simulink model "fcsystem"  (Simulink 5.0)
settings: Solver=ode23s  StartTime=0.0  StopTime=30.0  MaxStep=0.01  RelTol=1e-5
undefined symbols (not defined in the file or in its folder): alliedsignaleff, beta0, beta1, beta2, cm_kt, cm_kv, cm_maxtorque, cm_R, Cp, cp_inertia, dc, faradays, fc_activearea, fc_anode_volume, fc_cathode_volume, fc_inlet_flow_constant, fc_numberofcells, fc_outlet_flow_constant, fcx0, gamma, hydrogengasconstant, hydrogenmolarmass, im_volume, membranedrydensity, membranedryeqvweight, membranethickness, nitrogengasconstant, nitrogenmolarmass, om_At, om_Cd, om_outlet_choke_pr, om_volume, oxygengasconstant, oxygenmolarmass, phimax0, phimax1, phimax2, phimax3, phimax4, psimax0, psimax1, psimax2, psimax3, psimax4, psimax5, R, rho, Ta, universalgasconstant, vaporgasconstant, vapormolarmass
libraries: simulink x5
(part 2 of 3)

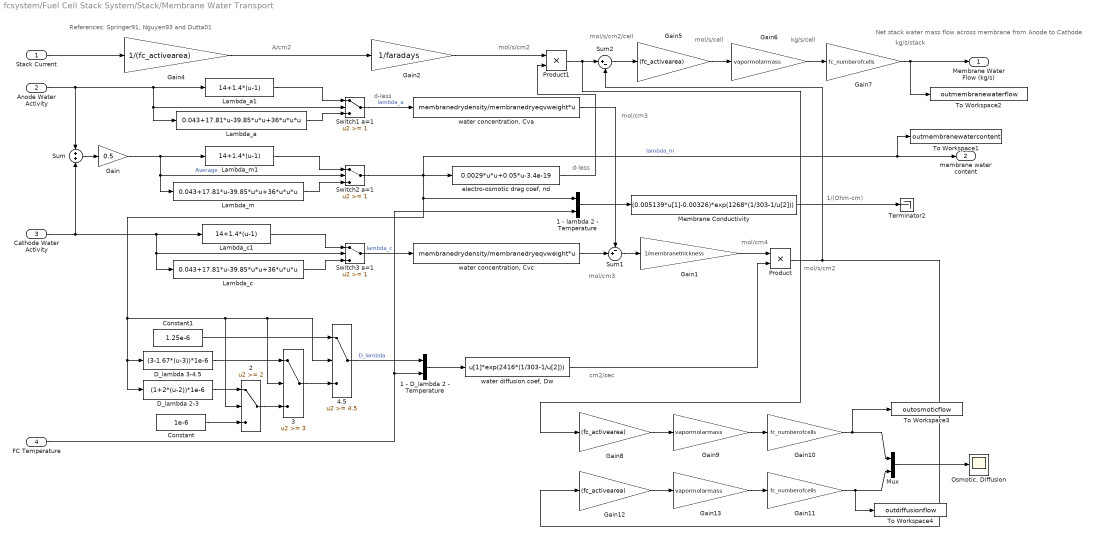
== system fcsystem/Fuel Cell Stack System/Stack/Membrane Water Transport ==
  note: kg/s/stack
  note: kg/s/cell
  note: mol/s/cell
  note: 1/(Ohm-cm)
  note: A/cm2
  note: mol/s/cm2/cell
  note: mol/s/cm2
  note: d-less
  note: mol/cm4
  note: cm2/sec
  note: mol/s/cm2
  note: mol/cm3
  note: mol/cm3
  note: d-less
  note: References: Springer91, Nguyen93 and Dutta01
  note: Net stack water mass flow
      | across membrane
      | from Anode to Cathode
  Stack Current : Inport
  Anode Water Activity : Inport  Port=2
  Cathode Water Activity : Inport  Port=3
  FC Temperature : Inport  Port=4
  1 - D_lambda 2 - Temperature : Mux  Inputs=2
  1 - lambda 2 - Temperature : Mux  Inputs=2
  2 : Switch  Threshold=2  SaturateOnIntegerOverflow=on  InputSameDT=on
  3 : Switch  Threshold=3  SaturateOnIntegerOverflow=on  InputSameDT=on
  4.5 : Switch  Threshold=4.5  SaturateOnIntegerOverflow=on  InputSameDT=on
  Constant : Constant  Value=1e-6
  Constant1 : Constant  Value=1.25e-6
  D_lambda 2-3 : Fcn  Expr=(1+2*(u-2))*1e-6
  D_lambda 3-4.5 : Fcn  Expr=(3-1.67*(u-3))*1e-6
  Gain : Gain  Gain=0.5  SaturateOnIntegerOverflow=on
  Gain1 : Gain  Gain=1/membranethickness  SaturateOnIntegerOverflow=on
  Gain10 : Gain  Gain=fc_numberofcells  SaturateOnIntegerOverflow=on
  Gain11 : Gain  Gain=fc_numberofcells  SaturateOnIntegerOverflow=on
  Gain12 : Gain  Gain=(fc_activearea)  SaturateOnIntegerOverflow=on
  Gain13 : Gain  Gain=vapormolarmass  SaturateOnIntegerOverflow=on
  Gain2 : Gain  Gain=1/faradays  SaturateOnIntegerOverflow=on
  Gain4 : Gain  Gain=1/(fc_activearea)  SaturateOnIntegerOverflow=on
  Gain5 : Gain  Gain=(fc_activearea)  SaturateOnIntegerOverflow=on
  Gain6 : Gain  Gain=vapormolarmass  SaturateOnIntegerOverflow=on
  Gain7 : Gain  Gain=fc_numberofcells  SaturateOnIntegerOverflow=on
  Gain8 : Gain  Gain=(fc_activearea)  SaturateOnIntegerOverflow=on
  Gain9 : Gain  Gain=vapormolarmass  SaturateOnIntegerOverflow=on
  Lambda_a : Fcn  Expr=0.043+17.81*u-39.85*u*u+36*u*u*u
  Lambda_a1 : Fcn  Expr=14+1.4*(u-1)
  Lambda_c : Fcn  Expr=0.043+17.81*u-39.85*u*u+36*u*u*u
  Lambda_c1 : Fcn  Expr=14+1.4*(u-1)
  Lambda_m : Fcn  Expr=0.043+17.81*u-39.85*u*u+36*u*u*u
  Lambda_m1 : Fcn  Expr=14+1.4*(u-1)
  Membrane Conductivity : Fcn  Expr=(0.005139*u[1]-0.00326)*exp(1268*(1/303-1/u[2]))
  Mux : Mux  Inputs=2
  "Osmotic, Diffusion" : Scope
      settings: TimeRange=15  YMin=0  YMax=0.02
  Product : Product  SaturateOnIntegerOverflow=on  InputSameDT=on
  Product1 : Product  SaturateOnIntegerOverflow=on  InputSameDT=on
  Sum : Sum  Inputs=+|+  SaturateOnIntegerOverflow=on  InputSameDT=on
  Sum1 : Sum  Inputs=-+|  SaturateOnIntegerOverflow=on  InputSameDT=on
  Sum2 : Sum  Inputs=|+-  SaturateOnIntegerOverflow=on  InputSameDT=on
  Switch1 a=1 : Switch  Threshold=1  SaturateOnIntegerOverflow=on  InputSameDT=on
  Switch2 a=1 : Switch  Threshold=1  SaturateOnIntegerOverflow=on  InputSameDT=on
  Switch3 a=1 : Switch  Threshold=1  SaturateOnIntegerOverflow=on  InputSameDT=on
  Terminator2 : Terminator
  To Workspace1 : ToWorkspace  VariableName=outmembranewatercontent  SampleTime=-1  SaveFormat=Array
  To Workspace2 : ToWorkspace  VariableName=outmembranewaterflow  SampleTime=-1  SaveFormat=Array
  To Workspace3 : ToWorkspace  VariableName=outosmoticflow  SampleTime=-1  SaveFormat=Array
  To Workspace4 : ToWorkspace  VariableName=outdiffusionflow  SampleTime=-1  SaveFormat=Array
  "electro-osmotic drag coef, nd" : Fcn  Expr=0.0029*u*u+0.05*u-3.4e-19
  "water concentration, Cva" : Fcn  Expr=membranedrydensity/membranedryeqvweight*u
  "water concentration, Cvc" : Fcn  Expr=membranedrydensity/membranedryeqvweight*u
  "water diffusion coef, Dw" : Fcn  Expr=u[1]*exp(2416*(1/303-1/u[2]))
  Membrane Water Flow (kg/s) : Outport
  membrane water content : Outport  Port=2
  wires:
  Gain11/1 -> To Workspace4/1, Mux/2
  Gain10/1 -> To Workspace3/1, Mux/1
  Gain7/1 -> To Workspace2/1, Membrane Water Flow (kg/s)/1
  Mux/1 -> "Osmotic, Diffusion"/1
  Product/1 -> Gain12/1, Sum2/2
  Gain13/1 -> Gain11/1
  Gain12/1 -> Gain13/1
  Gain9/1 -> Gain10/1
  Gain8/1 -> Gain9/1
  Product1/1 -> Gain8/1, Sum2/1
  Gain6/1 -> Gain7/1
  Gain5/1 -> Gain6/1
  Sum2/1 -> Gain5/1
  "electro-osmotic drag coef, nd"/1 -> Product1/2
  Gain2/1 -> Product1/1
  Gain4/1 -> Gain2/1
  Stack Current/1 -> Gain4/1
  1 - lambda 2 - Temperature/1 -> Membrane Conductivity/1
  FC Temperature/1 -> 1 - lambda 2 - Temperature/2, 1 - D_lambda 2 - Temperature/2
  Membrane Conductivity/1 -> Terminator2/1
  1 - D_lambda 2 - Temperature/1 -> "water diffusion coef, Dw"/1
  Gain1/1 -> Product/1
  "water diffusion coef, Dw"/1 -> Product/2
  Sum1/1 -> Gain1/1
  "water concentration, Cva"/1 -> Sum1/1
  "water concentration, Cvc"/1 -> Sum1/2
  Switch3 a=1/1 -> "water concentration, Cvc"/1  "lambda_c"
  Switch1 a=1/1 -> "water concentration, Cva"/1  "lambda_a"
  4.5/1 -> 1 - D_lambda 2 - Temperature/1  "D_lambda"
  Constant1/1 -> 4.5/1
  3/1 -> 4.5/3
  D_lambda 3-4.5/1 -> 3/1
  2/1 -> 3/3
  D_lambda 2-3/1 -> 2/1
  Lambda_c1/1 -> Switch3 a=1/1
  Lambda_c/1 -> Switch3 a=1/3
  Cathode Water Activity/1 -> Lambda_c/1, Switch3 a=1/2, Lambda_c1/1, Sum/2
  Constant/1 -> 2/3
  Switch2 a=1/1 -> To Workspace1/1, membrane water content/1, 1 - lambda 2 - Temperature/1, D_lambda 3-4.5/1, D_lambda 2-3/1, 2/2, 3/2, 4.5/2, "electro-osmotic drag coef, nd"/1  "lambda_m"
  Lambda_m/1 -> Switch2 a=1/3
  Lambda_m1/1 -> Switch2 a=1/1
  Gain/1 -> Lambda_m/1, Switch2 a=1/2, Lambda_m1/1  "Average"
  Sum/1 -> Gain/1
  Lambda_a/1 -> Switch1 a=1/3
  Lambda_a1/1 -> Switch1 a=1/1
  Anode Water Activity/1 -> Switch1 a=1/2, Lambda_a/1, Lambda_a1/1, Sum/1

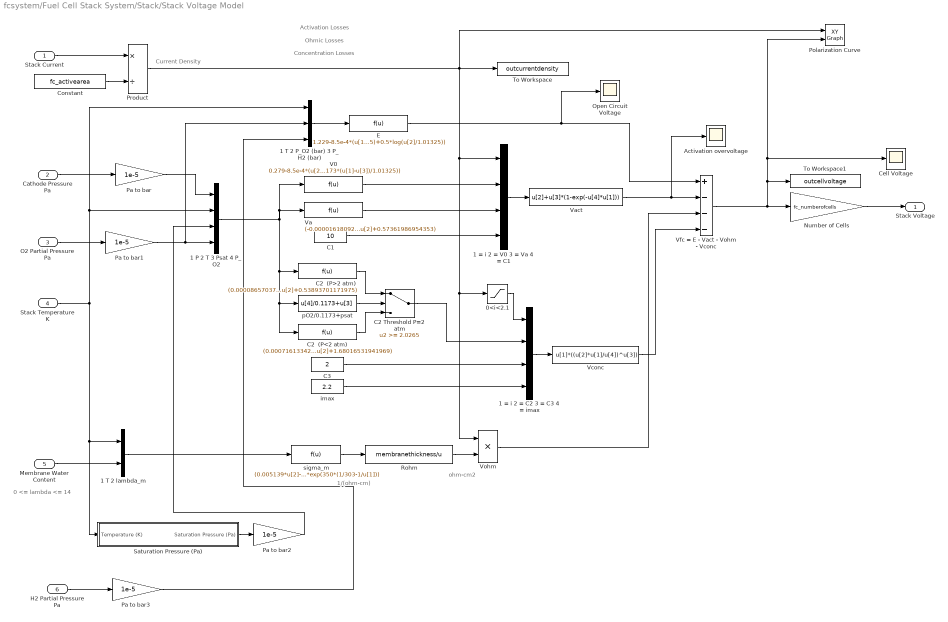
== system fcsystem/Fuel Cell Stack System/Stack/Stack Voltage Model ==
  note: Current Density
  note: 0 <= lambda <= 14
  note: 1/(ohm-cm)
  note: ohm-cm2
  note: Activation Losses
  note: Ohmic Losses
  note: Concentration Losses
  Stack Current : Inport
  Cathode Pressure Pa : Inport  Port=2
  O2 Partial Pressure Pa : Inport  Port=3
  Stack Temperature K : Inport  Port=4
  Membrane Water Content : Inport  Port=5
  H2 Partial Pressure Pa : Inport  Port=6
  0<i<2.1 : Saturate  UpperLimit=2.1  LowerLimit=0
  1 = i 2 = C2 3 = C3 4 = imax : Mux
  1 = i 2 = V0 3 = Va 4 = C1 : Mux
  1 P 2 T 3 Psat 4 P_O2 : Mux
  1 T 2 P_O2 (bar) 3 P_H2 (bar) : Mux  Inputs=3
  1 T 2 lambda_m : Mux  Inputs=2
  Activation overvoltage : Scope
      settings: TimeRange=15  YMin=0.425  YMax=0.455
  C1 : Constant  Value=10
  C2 Threshold P=2 atm : Switch  Threshold=2.0265  SaturateOnIntegerOverflow=on  InputSameDT=on
  C2  (P<2 atm) : Fcn  Expr=(0.00071613342996*u[2]-0.62205579736909)*(u[4]/0.1173+u[3])+(-0.00145360512618*u[2]+1.68016531941969)
  C2  (P>2 atm) : Fcn  Expr=(0.00008657037473*u[2]-0.06804881673615)*(u[4]/0.1173+u[3])+(-0.00015956699340*u[2]+0.53893701171975)
  C3 : Constant  Value=2
  Cell Voltage : Scope
      settings: TimeRange=15  YMin=0.62  YMax=0.68
  Constant : Constant  Value=fc_activearea
  E : Fcn  Expr=1.229-8.5e-4*(u[1]-298.15)+4.308e-5*u[1]*(log(u[3]/1.01325)+0.5*log(u[2]/1.01325))
  Number of Cells : Gain  Gain=fc_numberofcells  SaturateOnIntegerOverflow=on
  Open Circuit Voltage : Scope
      settings: TimeRange=15  YMin=1.17  YMax=1.185
  Pa to bar{,1..3} (4 alike) : Gain  Gain=1e-5  SaturateOnIntegerOverflow=on
  Polarization Curve : simulink/Sinks/XY Graph  xmin=0  xmax=2  ymin=0  ymax=1.3  st=-1
  Product : Product  Inputs=*/  SaturateOnIntegerOverflow=on  InputSameDT=on
  Rohm : Fcn  Expr=membranethickness/u
  Saturation Pressure (Pa) : Subsystem
  To Workspace : ToWorkspace  VariableName=outcurrentdensity  SampleTime=-1  SaveFormat=Array
  To Workspace1 : ToWorkspace  VariableName=outcellvoltage  SampleTime=-1  SaveFormat=Array
  V0 : Fcn  Expr=0.279-8.5e-4*(u[2]-298.15)+4.308e-5*u[2]*(log((u[1]-u[3])/1.01325)+0.5*log(0.1173*(u[1]-u[3])/1.01325))
  Va : Fcn  Expr=(-0.00001618092702*u[2]+0.01617607122728)*(u[4]/0.1173+u[3])^2+(0.00018055303614*u[2]-0.16636610322644)*(u[4]/0.1173+u[3])+(-0.00058195751420*u[2]+0.57361986954353)
  Vact : Fcn  Expr=u[2]+u[3]*(1-exp(-u[4]*u[1]))
  Vconc : Fcn  Expr=u[1]*((u[2]*u[1]/u[4])^u[3])
  Vfc = E - Vact - Vohm - Vconc : Sum  Inputs=+---  SaturateOnIntegerOverflow=on  InputSameDT=on
  Vohm : Product  SaturateOnIntegerOverflow=on  InputSameDT=on
  imax : Constant  Value=2.2
  pO2/0.1173+psat : Fcn  Expr=u[4]/0.1173+u[3]
  sigma_m : Fcn  Expr=(0.005139*u[2]-0.00326)*exp(350*(1/303-1/u[1]))
  Stack Voltage : Outport
  wires:
  Vfc = E - Vact - Vohm - Vconc/1 -> Number of Cells/1, Cell Voltage/1, Polarization Curve/2, To Workspace1/1
  Number of Cells/1 -> Stack Voltage/1
  Vconc/1 -> Vfc = E - Vact - Vohm - Vconc/4
  Vohm/1 -> Vfc = E - Vact - Vohm - Vconc/3
  Vact/1 -> Vfc = E - Vact - Vohm - Vconc/2, Activation overvoltage/1
  Stack Current/1 -> Product/1
  Constant/1 -> Product/2
  O2 Partial Pressure Pa/1 -> Pa to bar1/1
  Stack Temperature K/1 -> 1 P 2 T 3 Psat 4 P_O2/2, 1 T 2 P_O2 (bar) 3 P_H2 (bar)/1, Saturation Pressure (Pa)/1(Temperature (K)), 1 T 2 lambda_m/1
  1 T 2 P_O2 (bar) 3 P_H2 (bar)/1 -> E/1
  1 P 2 T 3 Psat 4 P_O2/1 -> V0/1, Va/1, C2  (P<2 atm)/1, pO2/0.1173+psat/1, C2  (P>2 atm)/1
  Saturation Pressure (Pa)/1(Saturation Pressure (Pa)) -> Pa to bar2/1
  C1/1 -> 1 = i 2 = V0 3 = Va 4 = C1/4
  Va/1 -> 1 = i 2 = V0 3 = Va 4 = C1/3
  1 = i 2 = C2 3 = C3 4 = imax/1 -> Vconc/1
  C2 Threshold P=2 atm/1 -> 1 = i 2 = C2 3 = C3 4 = imax/2
  C3/1 -> 1 = i 2 = C2 3 = C3 4 = imax/3
  imax/1 -> 1 = i 2 = C2 3 = C3 4 = imax/4
  0<i<2.1/1 -> 1 = i 2 = C2 3 = C3 4 = imax/1
  Cathode Pressure Pa/1 -> Pa to bar/1
  Pa to bar1/1 -> 1 P 2 T 3 Psat 4 P_O2/4, 1 T 2 P_O2 (bar) 3 P_H2 (bar)/2
  Membrane Water Content/1 -> 1 T 2 lambda_m/2
  1 T 2 lambda_m/1 -> sigma_m/1
  sigma_m/1 -> Rohm/1
  Rohm/1 -> Vohm/2
  Product/1 -> 1 = i 2 = V0 3 = Va 4 = C1/1, 0<i<2.1/1, Vohm/1, To Workspace/1, Polarization Curve/1
  C2  (P>2 atm)/1 -> C2 Threshold P=2 atm/1
  C2  (P<2 atm)/1 -> C2 Threshold P=2 atm/3
  pO2/0.1173+psat/1 -> C2 Threshold P=2 atm/2
  1 = i 2 = V0 3 = Va 4 = C1/1 -> Vact/1
  E/1 -> Open Circuit Voltage/1, Vfc = E - Vact - Vohm - Vconc/1
  V0/1 -> 1 = i 2 = V0 3 = Va 4 = C1/2
  Pa to bar/1 -> 1 P 2 T 3 Psat 4 P_O2/1
  Pa to bar2/1 -> 1 P 2 T 3 Psat 4 P_O2/3
  H2 Partial Pressure Pa/1 -> Pa to bar3/1
  Pa to bar3/1 -> 1 T 2 P_O2 (bar) 3 P_H2 (bar)/3

== system fcsystem/Fuel Cell Stack System/Static Humidifier/Saturation Pressure (Pa) ==
  Temperature (K) : Inport
  333.15K : Switch  Threshold=333.15  SaturateOnIntegerOverflow=on  InputSameDT=on
  433.15K : Switch  Threshold=433.15  SaturateOnIntegerOverflow=on  InputSameDT=on
  533.15K : Switch  Threshold=533.15  SaturateOnIntegerOverflow=on  InputSameDT=on
  Display{3..7} (5 alike) : Display
  Water Sat. Pressure in kPa (using 4th order approx) 333.15K<t<433.15K : Fcn  Expr=1.508306069874139e-006*u^4-0.00184416225407*u^3+0.85777718452468*u^2-1.796665242102233e+002*u+1.428163901107325e+004
  Water Sat. Pressure in kPa (using 4th order approx) 433.15<t<533.15 : Fcn  Expr=1.338811201296496e-006*u^4-0.00154136533415*u^3+0.65477998701526*u^2-1.191331991860853e+002*u+7.506492157825003e+003
  Water Sat. Pressure in kPa (using 4th order approx) t<333.15K : Fcn  Expr=6.853193243616891e-007*u^4-7.432459524835483e-004*u^3+0.30413751828818*u^2-55.61363113326989*u+3.831800671740628e+003
  Water Sat. Pressure in kPa (using 4th order approx) t>533.15K : Fcn  Expr=1.648503329422670e-6*u^4-0.00209262218193*u^3+1.01793196387371*u^2-2.241752317908023e2*u+1.878246444328017e4
  kPa to Pa : Gain  Gain=1000  SaturateOnIntegerOverflow=on
  Saturation Pressure (Pa) : Outport
  wires:
  Temperature (K)/1 -> Water Sat. Pressure in kPa (using 4th order approx) t>533.15K/1, Water Sat. Pressure in kPa (using 4th order approx) 433.15<t<533.15/1, Water Sat. Pressure in kPa (using 4th order approx) 333.15K<t<433.15K/1, Water Sat. Pressure in kPa (using 4th order approx) t<333.15K/1, 533.15K/2, 433.15K/2, 333.15K/2
  Water Sat. Pressure in kPa (using 4th order approx) t>533.15K/1 -> 533.15K/1
  Water Sat. Pressure in kPa (using 4th order approx) 433.15<t<533.15/1 -> 433.15K/1
  Water Sat. Pressure in kPa (using 4th order approx) 333.15K<t<433.15K/1 -> 333.15K/1
  333.15K/1 -> 433.15K/3, Display3/1
  433.15K/1 -> 533.15K/3, Display4/1
  533.15K/1 -> kPa to Pa/1, Display5/1
  Water Sat. Pressure in kPa (using 4th order approx) t<333.15K/1 -> 333.15K/3, Display6/1
  kPa to Pa/1 -> Saturation Pressure (Pa)/1, Display7/1

== system fcsystem/Fuel Cell Stack System/Compressor/Compressor/Calculate Humidity Change ==
  note: Pv2 = (P2/P1)*Pv1
      | Pa2 = (P2/P1)*Pa1
      | phi2 = Pv2/Psat(T2) = P2*Pv1/P1/Psat(T2) = P2*phi1*Psat(T1)/P1/Psat(T2)
  Pressure 1 : Inport
  Pressure 2 : Inport  Port=2
  Temperature 1 : Inport  Port=3
  Temperature 2 : Inport  Port=4
  Humidity 1 : Inport  Port=5
  Product : Product  Inputs=***//  SaturateOnIntegerOverflow=on  InputSameDT=on
  Saturation 0-1 : Saturate  UpperLimit=1  LowerLimit=0
  Saturation Pressure (Pa) : Subsystem
  Saturation Pressure (Pa)1 : Subsystem
  Humidity 2 : Outport
  wires:
  Temperature 2/1 -> Saturation Pressure (Pa)1/1(Temperature (K))
  Humidity 1/1 -> Product/2
  Pressure 2/1 -> Product/1
  Pressure 1/1 -> Product/4
  Temperature 1/1 -> Saturation Pressure (Pa)/1(Temperature (K))
  Saturation Pressure (Pa)1/1(Saturation Pressure (Pa)) -> Product/5
  Saturation Pressure (Pa)/1(Saturation Pressure (Pa)) -> Product/3
  Product/1 -> Saturation 0-1/1
  Saturation 0-1/1 -> Humidity 2/1

== system fcsystem/Fuel Cell Stack System/Compressor/Compressor/Compressor  Map ==
  note: Pressure Ratio at Zero Flow
  note: lb/min
  Pressure Ratio In : Inport
  Corrected Speed (rpm) : Inport  Port=2
  Compressor Efficiency : Subsystem
  Constant : Constant  Value=0
  Constant1 : Constant  Value=1000
  Gain : Gain  Gain=1/100  SaturateOnIntegerOverflow=on
  Jensen&Kristensen Compressor Map : Subsystem
  Max Pressure Ratio : MinMax  Inputs=2
  Min Pressure Ratio : MinMax  Function=max  Inputs=2
  kg/sec to lb/min : Gain  Gain=132.2775  SaturateOnIntegerOverflow=on
  Corrected Air Flow : Outport
  Efficiency : Outport  Port=2
  Pressure Ratio Out : Outport  Port=3
  wires:
  Gain/1 -> Efficiency/1
  Corrected Speed (rpm)/1 -> Jensen&Kristensen Compressor Map/2(Corrected Speed (rpm))
  Constant1/1 -> Max Pressure Ratio/2
  Max Pressure Ratio/1 -> Pressure Ratio Out/1, Jensen&Kristensen Compressor Map/1(Pressure Ratio), Compressor Efficiency/2(Pressure Ratio)
  Min Pressure Ratio/1 -> Max Pressure Ratio/1
  Constant/1 -> Min Pressure Ratio/2
  Pressure Ratio In/1 -> Min Pressure Ratio/1
  Compressor Efficiency/1(Efficiency) -> Gain/1
  kg/sec to lb/min/1 -> Compressor Efficiency/1(Flow lb/min)
  Jensen&Kristensen Compressor Map/1(Air Flow (kg/sec)) -> Corrected Air Flow/1, kg/sec to lb/min/1

== system fcsystem/Fuel Cell Stack System/Inlet Manifold/Calculate Humidity Change/Saturation Pressure (Pa) ==
  Temperature (K) : Inport
  333.15K : Switch  Threshold=333.15  SaturateOnIntegerOverflow=on  InputSameDT=on
  433.15K : Switch  Threshold=433.15  SaturateOnIntegerOverflow=on  InputSameDT=on
  533.15K : Switch  Threshold=533.15  SaturateOnIntegerOverflow=on  InputSameDT=on
  Water Sat. Pressure in kPa (using 4th order approx) 333.15K<t<433.15K : Fcn  Expr=1.508306069874139e-006*u^4-0.00184416225407*u^3+0.85777718452468*u^2-1.796665242102233e+002*u+1.428163901107325e+004
  Water Sat. Pressure in kPa (using 4th order approx) 433.15<t<533.15 : Fcn  Expr=1.338811201296496e-006*u^4-0.00154136533415*u^3+0.65477998701526*u^2-1.191331991860853e+002*u+7.506492157825003e+003
  Water Sat. Pressure in kPa (using 4th order approx) t<333.15K : Fcn  Expr=6.853193243616891e-007*u^4-7.432459524835483e-004*u^3+0.30413751828818*u^2-55.61363113326989*u+3.831800671740628e+003
  Water Sat. Pressure in kPa (using 4th order approx) t>533.15K : Fcn  Expr=1.648503329422670e-6*u^4-0.00209262218193*u^3+1.01793196387371*u^2-2.241752317908023e2*u+1.878246444328017e4
  kPa to Pa : Gain  Gain=1000  SaturateOnIntegerOverflow=on
  Saturation Pressure (Pa) : Outport
  wires:
  Water Sat. Pressure in kPa (using 4th order approx) t<333.15K/1 -> 333.15K/3
  Water Sat. Pressure in kPa (using 4th order approx) 333.15K<t<433.15K/1 -> 333.15K/1
  333.15K/1 -> 433.15K/3
  Water Sat. Pressure in kPa (using 4th order approx) 433.15<t<533.15/1 -> 433.15K/1
  Water Sat. Pressure in kPa (using 4th order approx) t>533.15K/1 -> 533.15K/1
  433.15K/1 -> 533.15K/3
  kPa to Pa/1 -> Saturation Pressure (Pa)/1
  533.15K/1 -> kPa to Pa/1
  Temperature (K)/1 -> 333.15K/2, 433.15K/2, 533.15K/2, Water Sat. Pressure in kPa (using 4th order approx) t<333.15K/1, Water Sat. Pressure in kPa (using 4th order approx) 333.15K<t<433.15K/1, Water Sat. Pressure in kPa (using 4th order approx) 433.15<t<533.15/1, Water Sat. Pressure in kPa (using 4th order approx) t>533.15K/1

== system fcsystem/Fuel Cell Stack System/Inlet Manifold/Calculate Humidity Change/Saturation Pressure (Pa)1 ==
  Temperature (K) : Inport
  333.15K : Switch  Threshold=333.15  SaturateOnIntegerOverflow=on  InputSameDT=on
  433.15K : Switch  Threshold=433.15  SaturateOnIntegerOverflow=on  InputSameDT=on
  533.15K : Switch  Threshold=533.15  SaturateOnIntegerOverflow=on  InputSameDT=on
  Display{1..5} (5 alike) : Display
  Water Sat. Pressure in kPa (using 4th order approx) 333.15K<t<433.15K : Fcn  Expr=1.508306069874139e-006*u^4-0.00184416225407*u^3+0.85777718452468*u^2-1.796665242102233e+002*u+1.428163901107325e+004
  Water Sat. Pressure in kPa (using 4th order approx) 433.15<t<533.15 : Fcn  Expr=1.338811201296496e-006*u^4-0.00154136533415*u^3+0.65477998701526*u^2-1.191331991860853e+002*u+7.506492157825003e+003
  Water Sat. Pressure in kPa (using 4th order approx) t<333.15K : Fcn  Expr=6.853193243616891e-007*u^4-7.432459524835483e-004*u^3+0.30413751828818*u^2-55.61363113326989*u+3.831800671740628e+003
  Water Sat. Pressure in kPa (using 4th order approx) t>533.15K : Fcn  Expr=1.648503329422670e-6*u^4-0.00209262218193*u^3+1.01793196387371*u^2-2.241752317908023e2*u+1.878246444328017e4
  kPa to Pa : Gain  Gain=1000  SaturateOnIntegerOverflow=on
  Saturation Pressure (Pa) : Outport
  wires:
  kPa to Pa/1 -> Saturation Pressure (Pa)/1
  Water Sat. Pressure in kPa (using 4th order approx) t>533.15K/1 -> 533.15K/1
  Water Sat. Pressure in kPa (using 4th order approx) 433.15<t<533.15/1 -> 433.15K/1
  Water Sat. Pressure in kPa (using 4th order approx) 333.15K<t<433.15K/1 -> 333.15K/1
  333.15K/1 -> 433.15K/3, Display1/1
  433.15K/1 -> 533.15K/3, Display2/1
  Water Sat. Pressure in kPa (using 4th order approx) t<333.15K/1 -> 333.15K/3, Display3/1
  533.15K/1 -> kPa to Pa/1, Display4/1
  Temperature (K)/1 -> Water Sat. Pressure in kPa (using 4th order approx) t>533.15K/1, Water Sat. Pressure in kPa (using 4th order approx) 433.15<t<533.15/1, Water Sat. Pressure in kPa (using 4th order approx) 333.15K<t<433.15K/1, Water Sat. Pressure in kPa (using 4th order approx) t<333.15K/1, 533.15K/2, 433.15K/2, 333.15K/2, Display5/1

== system fcsystem/Fuel Cell Stack System/Magic Cooler/Calculate Humidity Change/Saturation Pressure (Pa) ==
  Temperature (K) : Inport
  333.15K : Switch  Threshold=333.15  SaturateOnIntegerOverflow=on  InputSameDT=on
  433.15K : Switch  Threshold=433.15  SaturateOnIntegerOverflow=on  InputSameDT=on
  533.15K : Switch  Threshold=533.15  SaturateOnIntegerOverflow=on  InputSameDT=on
  Water Sat. Pressure in kPa (using 4th order approx) 333.15K<t<433.15K : Fcn  Expr=1.508306069874139e-006*u^4-0.00184416225407*u^3+0.85777718452468*u^2-1.796665242102233e+002*u+1.428163901107325e+004
  Water Sat. Pressure in kPa (using 4th order approx) 433.15<t<533.15 : Fcn  Expr=1.338811201296496e-006*u^4-0.00154136533415*u^3+0.65477998701526*u^2-1.191331991860853e+002*u+7.506492157825003e+003
  Water Sat. Pressure in kPa (using 4th order approx) t<333.15K : Fcn  Expr=6.853193243616891e-007*u^4-7.432459524835483e-004*u^3+0.30413751828818*u^2-55.61363113326989*u+3.831800671740628e+003
  Water Sat. Pressure in kPa (using 4th order approx) t>533.15K : Fcn  Expr=1.648503329422670e-6*u^4-0.00209262218193*u^3+1.01793196387371*u^2-2.241752317908023e2*u+1.878246444328017e4
  kPa to Pa : Gain  Gain=1000  SaturateOnIntegerOverflow=on
  Saturation Pressure (Pa) : Outport
  wires:
  Water Sat. Pressure in kPa (using 4th order approx) t<333.15K/1 -> 333.15K/3
  Water Sat. Pressure in kPa (using 4th order approx) 333.15K<t<433.15K/1 -> 333.15K/1
  333.15K/1 -> 433.15K/3
  Water Sat. Pressure in kPa (using 4th order approx) 433.15<t<533.15/1 -> 433.15K/1
  Water Sat. Pressure in kPa (using 4th order approx) t>533.15K/1 -> 533.15K/1
  433.15K/1 -> 533.15K/3
  kPa to Pa/1 -> Saturation Pressure (Pa)/1
  533.15K/1 -> kPa to Pa/1
  Temperature (K)/1 -> 333.15K/2, 433.15K/2, 533.15K/2, Water Sat. Pressure in kPa (using 4th order approx) t<333.15K/1, Water Sat. Pressure in kPa (using 4th order approx) 333.15K<t<433.15K/1, Water Sat. Pressure in kPa (using 4th order approx) 433.15<t<533.15/1, Water Sat. Pressure in kPa (using 4th order approx) t>533.15K/1

== system fcsystem/Fuel Cell Stack System/Magic Cooler/Calculate Humidity Change/Saturation Pressure (Pa)1 ==
  Temperature (K) : Inport
  333.15K : Switch  Threshold=333.15  SaturateOnIntegerOverflow=on  InputSameDT=on
  433.15K : Switch  Threshold=433.15  SaturateOnIntegerOverflow=on  InputSameDT=on
  533.15K : Switch  Threshold=533.15  SaturateOnIntegerOverflow=on  InputSameDT=on
  Display{1..5} (5 alike) : Display
  Water Sat. Pressure in kPa (using 4th order approx) 333.15K<t<433.15K : Fcn  Expr=1.508306069874139e-006*u^4-0.00184416225407*u^3+0.85777718452468*u^2-1.796665242102233e+002*u+1.428163901107325e+004
  Water Sat. Pressure in kPa (using 4th order approx) 433.15<t<533.15 : Fcn  Expr=1.338811201296496e-006*u^4-0.00154136533415*u^3+0.65477998701526*u^2-1.191331991860853e+002*u+7.506492157825003e+003
  Water Sat. Pressure in kPa (using 4th order approx) t<333.15K : Fcn  Expr=6.853193243616891e-007*u^4-7.432459524835483e-004*u^3+0.30413751828818*u^2-55.61363113326989*u+3.831800671740628e+003
  Water Sat. Pressure in kPa (using 4th order approx) t>533.15K : Fcn  Expr=1.648503329422670e-6*u^4-0.00209262218193*u^3+1.01793196387371*u^2-2.241752317908023e2*u+1.878246444328017e4
  kPa to Pa : Gain  Gain=1000  SaturateOnIntegerOverflow=on
  Saturation Pressure (Pa) : Outport
  wires:
  kPa to Pa/1 -> Saturation Pressure (Pa)/1
  Water Sat. Pressure in kPa (using 4th order approx) t>533.15K/1 -> 533.15K/1
  Water Sat. Pressure in kPa (using 4th order approx) 433.15<t<533.15/1 -> 433.15K/1
  Water Sat. Pressure in kPa (using 4th order approx) 333.15K<t<433.15K/1 -> 333.15K/1
  333.15K/1 -> 433.15K/3, Display1/1
  433.15K/1 -> 533.15K/3, Display2/1
  Water Sat. Pressure in kPa (using 4th order approx) t<333.15K/1 -> 333.15K/3, Display3/1
  533.15K/1 -> kPa to Pa/1, Display4/1
  Temperature (K)/1 -> Water Sat. Pressure in kPa (using 4th order approx) t>533.15K/1, Water Sat. Pressure in kPa (using 4th order approx) 433.15<t<533.15/1, Water Sat. Pressure in kPa (using 4th order approx) 333.15K<t<433.15K/1, Water Sat. Pressure in kPa (using 4th order approx) t<333.15K/1, 533.15K/2, 433.15K/2, 333.15K/2, Display5/1

== system fcsystem/Fuel Cell Stack System/Stack/Anode Mass Flow Model/Hydrogen Balance ==
  H2 Mass Flow In (kg/s) : Inport
  H2 Mass Flow out (kg/s) : Inport  Port=2
  H2 Mass reacted (kg/s) : Inport  Port=3
  FC Temperature (K) : Inport  Port=4
  Initial Condition (kg) : Constant  Value=fcx0(2)
  Integrator : Integrator  InitialConditionSource=external
  Mux : Mux  Inputs=2
  Partial Pressure : Fcn  Expr=u[1]*hydrogengasconstant*u[2]/fc_anode_volume
  Product : Product  Inputs=*/  SaturateOnIntegerOverflow=on  InputSameDT=on
  Sum : Sum  Inputs=+--  SaturateOnIntegerOverflow=on  InputSameDT=on
  H2 Mass (kg) : Outport
  H2 Partial Pressure : Outport  Port=2
  H2 Excess Ratio : Outport  Port=3
  tag scope: mH2=global
  wires:
  Product/1 -> H2 Excess Ratio/1
  H2 Mass reacted (kg/s)/1 -> Product/2, Sum/3
  H2 Mass Flow out (kg/s)/1 -> Sum/2
  H2 Mass Flow In (kg/s)/1 -> Product/1, Sum/1
  Partial Pressure/1 -> H2 Partial Pressure/1
  Mux/1 -> Partial Pressure/1
  Integrator/1 -> Mux/1, H2 Mass (kg)/1, [mH2]
  FC Temperature (K)/1 -> Mux/2
  Initial Condition (kg)/1 -> Integrator/2
  Sum/1 -> Integrator/1

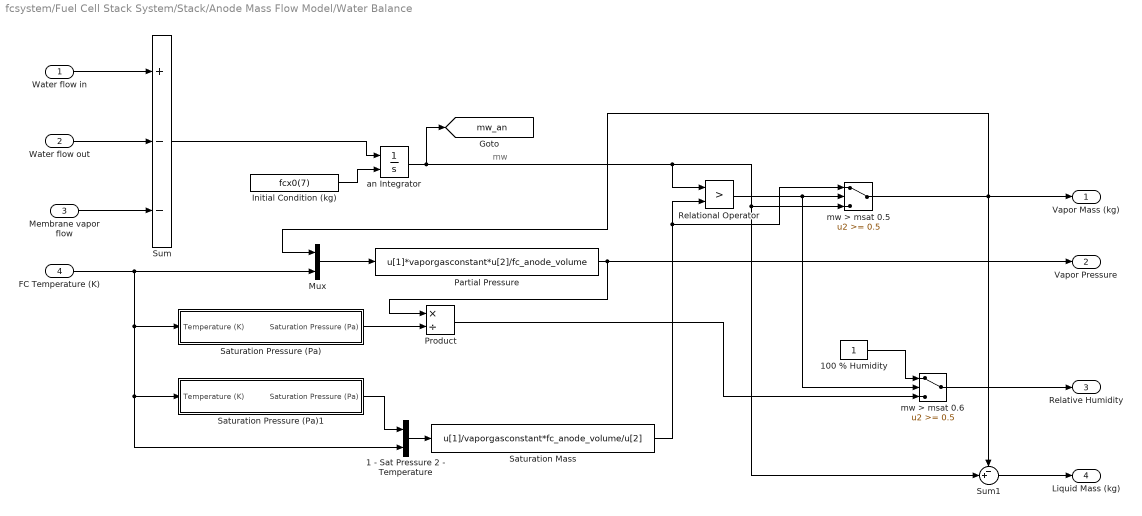
== system fcsystem/Fuel Cell Stack System/Stack/Anode Mass Flow Model/Water Balance ==
  note: mw
  Water flow in : Inport
  Water flow out : Inport  Port=2
  Membrane vapor flow : Inport  Port=3
  FC Temperature (K) : Inport  Port=4
  1 - Sat Pressure 2 - Temperature : Mux  Inputs=2
  100 % Humidity : Constant
  Initial Condition (kg) : Constant  Value=fcx0(7)
  Mux : Mux  Inputs=2
  Partial Pressure : Fcn  Expr=u[1]*vaporgasconstant*u[2]/fc_anode_volume
  Product : Product  Inputs=*/  SaturateOnIntegerOverflow=on  InputSameDT=on
  Relational Operator : RelationalOperator  Operator=>  InputSameDT=on
  Saturation Mass : Fcn  Expr=u[1]/vaporgasconstant*fc_anode_volume/u[2]
  Saturation Pressure (Pa) : Subsystem
  Saturation Pressure (Pa)1 : Subsystem
  Sum : Sum  Inputs=+--  SaturateOnIntegerOverflow=on  InputSameDT=on
  Sum1 : Sum  Inputs=-+|  SaturateOnIntegerOverflow=on  InputSameDT=on
  an Integrator : Integrator  InitialConditionSource=external
  mw > msat 0.5 : Switch  Threshold=0.5  SaturateOnIntegerOverflow=on  InputSameDT=on
  mw > msat 0.6 : Switch  Threshold=0.5  SaturateOnIntegerOverflow=on  InputSameDT=on
  Vapor Mass (kg) : Outport
  Vapor Pressure : Outport  Port=2
  Relative Humidity : Outport  Port=3
  Liquid Mass (kg) : Outport  Port=4
  tag scope: mw_an=global
  wires:
  an Integrator/1 -> Sum1/2, mw > msat 0.5/3, Relational Operator/1, [mw_an]
  Sum1/1 -> Liquid Mass (kg)/1
  mw > msat 0.5/1 -> Sum1/1, Mux/1, Vapor Mass (kg)/1
  mw > msat 0.6/1 -> Relative Humidity/1
  Product/1 -> mw > msat 0.6/3
  100 % Humidity/1 -> mw > msat 0.6/1
  Relational Operator/1 -> mw > msat 0.6/2, mw > msat 0.5/2
  Saturation Mass/1 -> mw > msat 0.5/1, Relational Operator/2
  1 - Sat Pressure 2 - Temperature/1 -> Saturation Mass/1
  Saturation Pressure (Pa)1/1(Saturation Pressure (Pa)) -> 1 - Sat Pressure 2 - Temperature/1
  Mux/1 -> Partial Pressure/1
  Partial Pressure/1 -> Vapor Pressure/1, Product/1
  Saturation Pressure (Pa)/1(Saturation Pressure (Pa)) -> Product/2
  Initial Condition (kg)/1 -> an Integrator/2
  Sum/1 -> an Integrator/1
  FC Temperature (K)/1 -> Saturation Pressure (Pa)1/1(Temperature (K)), 1 - Sat Pressure 2 - Temperature/2, Saturation Pressure (Pa)/1(Temperature (K)), Mux/2
  Membrane vapor flow/1 -> Sum/3
  Water flow out/1 -> Sum/2
  Water flow in/1 -> Sum/1

== system fcsystem/Fuel Cell Stack System/Stack/Anode Mass Flow Model/inlet flow properties to mass flow ==
  note: Units
      | Pressure - Pascal, bar
      | Temperature - Kelvin
      | Voltage - Volt
      | Current - Ampere
      | Mass Flow - kg/sec
      | Rotational Speed - rad/sec
      | Power - Watt
      | humidity or relative humidity - 0 to 1
  Anode Flow in : Inport
  1 - Total Mass Flow 2 - Temperature 3 - Pressure 4 - Relative Humidity : Demux
  Constant1 : Constant  Value=vapormolarmass/hydrogenmolarmass
  Constant2 : Constant
  Product2 : Product  SaturateOnIntegerOverflow=on  InputSameDT=on
  Product5 : Product  Inputs=*/  SaturateOnIntegerOverflow=on  InputSameDT=on
  Product6 : Product  SaturateOnIntegerOverflow=on  InputSameDT=on
  Product7 : Product  Inputs=*/  SaturateOnIntegerOverflow=on  InputSameDT=on
  Saturation Pressure (Pa) : Subsystem
  Sum4 : Sum  Inputs=-|+  SaturateOnIntegerOverflow=on  InputSameDT=on
  Sum5 : Sum  Inputs=++|  SaturateOnIntegerOverflow=on  InputSameDT=on
  Sum6 : Sum  Inputs=-+|  SaturateOnIntegerOverflow=on  InputSameDT=on
  To Workspace1 : ToWorkspace  VariableName=outANflowratein  SampleTime=-1  SaveFormat=Array
  Dry H2 Mass Flow in : Outport
  Vapor Mass Flow in : Outport  Port=2
  wires:
  1 - Total Mass Flow 2 - Temperature 3 - Pressure 4 - Relative Humidity/1 -> Product7/1, Sum6/2, To Workspace1/1
  Saturation Pressure (Pa)/1(Saturation Pressure (Pa)) -> Product2/1
  Product7/1 -> Dry H2 Mass Flow in/1, Sum6/1  "dry H2 mass flow"
  Sum6/1 -> Vapor Mass Flow in/1  "vapor mass flow"
  Constant2/1 -> Sum5/1
  Sum5/1 -> Product7/2
  Constant1/1 -> Product6/2
  Product6/1 -> Sum5/2  "Humidity Ratio"
  Product5/1 -> Product6/1
  Product2/1 -> Product5/1, Sum4/1  "vapor partial pressure"
  Sum4/1 -> Product5/2  "Dry H2 partial pressure"
  1 - Total Mass Flow 2 - Temperature 3 - Pressure 4 - Relative Humidity/3 -> Sum4/2
  1 - Total Mass Flow 2 - Temperature 3 - Pressure 4 - Relative Humidity/4 -> Product2/2
  1 - Total Mass Flow 2 - Temperature 3 - Pressure 4 - Relative Humidity/2 -> Saturation Pressure (Pa)/1(Temperature (K))
  Anode Flow in/1 -> 1 - Total Mass Flow 2 - Temperature 3 - Pressure 4 - Relative Humidity/1

== system fcsystem/Fuel Cell Stack System/Stack/Anode Mass Flow Model/outlet flow properties to mass flow ==
  note: Units
      | Pressure - Pascal, bar
      | Temperature - Kelvin
      | Voltage - Volt
      | Current - Ampere
      | Mass Flow - kg/sec
      | Rotational Speed - rad/sec
      | Power - Watt
      | humidity or relative humidity - 0 to 1
  Anode Flow out : Inport
  1 - Total Mass Flow 2 - Temperature 3 - Pressure 4 - Relative Humidity : Demux
  Constant1 : Constant  Value=vapormolarmass/hydrogenmolarmass
  Constant2 : Constant
  Product2 : Product  SaturateOnIntegerOverflow=on  InputSameDT=on
  Product5 : Product  Inputs=*/  SaturateOnIntegerOverflow=on  InputSameDT=on
  Product6 : Product  SaturateOnIntegerOverflow=on  InputSameDT=on
  Product7 : Product  Inputs=*/  SaturateOnIntegerOverflow=on  InputSameDT=on
  Saturation Pressure (Pa) : Subsystem
  Sum4 : Sum  Inputs=-|+  SaturateOnIntegerOverflow=on  InputSameDT=on
  Sum5 : Sum  Inputs=++|  SaturateOnIntegerOverflow=on  InputSameDT=on
  Sum6 : Sum  Inputs=-+|  SaturateOnIntegerOverflow=on  InputSameDT=on
  Dry H2 Mass Flow out : Outport
  Vapor Mass Flow out : Outport  Port=2
  wires:
  Anode Flow out/1 -> 1 - Total Mass Flow 2 - Temperature 3 - Pressure 4 - Relative Humidity/1
  1 - Total Mass Flow 2 - Temperature 3 - Pressure 4 - Relative Humidity/2 -> Saturation Pressure (Pa)/1(Temperature (K))
  Saturation Pressure (Pa)/1(Saturation Pressure (Pa)) -> Product2/1
  1 - Total Mass Flow 2 - Temperature 3 - Pressure 4 - Relative Humidity/4 -> Product2/2
  1 - Total Mass Flow 2 - Temperature 3 - Pressure 4 - Relative Humidity/3 -> Sum4/2
  Sum4/1 -> Product5/2  "Dry H2 partial pressure"
  Product2/1 -> Sum4/1, Product5/1  "vapor partial pressure"
  Product5/1 -> Product6/1
  Product6/1 -> Sum5/2  "Humidity Ratio"
  Constant1/1 -> Product6/2
  Sum5/1 -> Product7/2
  Constant2/1 -> Sum5/1
  1 - Total Mass Flow 2 - Temperature 3 - Pressure 4 - Relative Humidity/1 -> Product7/1, Sum6/2
  Sum6/1 -> Vapor Mass Flow out/1  "vapor mass flow"
  Product7/1 -> Sum6/1, Dry H2 Mass Flow out/1  "dry H2 mass flow"

== system fcsystem/Fuel Cell Stack System/Stack/Cathode Mass Flow Model/Cathode Exit Flow Rate ==
  Cathode Pressure : Inport
  OM Pressure : Inport  Port=2
  Gain : Gain  Gain=fc_outlet_flow_constant  SaturateOnIntegerOverflow=on
  Sum : Sum  Inputs=+|-  SaturateOnIntegerOverflow=on  InputSameDT=on
  Exit Flow Rate (kg/s) : Outport
  wires:
  Cathode Pressure/1 -> Sum/1
  OM Pressure/1 -> Sum/2
  Sum/1 -> Gain/1
  Gain/1 -> Exit Flow Rate (kg/s)/1

== system fcsystem/Fuel Cell Stack System/Stack/Cathode Mass Flow Model/Electrochemistry  Reaction ==
  Current : Inport
  O2 mass flow in : Inport  Port=2
  Stack Voltage : Inport  Port=3
  1/n : Gain  Gain=1/fc_numberofcells  SaturateOnIntegerOverflow=on
  Ideal Cell Voltage : Constant  Description=See larminie page 25 and 27  Value=1.25
  Oxygen Molar Mass : Gain  Gain=32e-3  SaturateOnIntegerOverflow=on
  Product : Product  Inputs=*/  SaturateOnIntegerOverflow=on  InputSameDT=on
  Product1 : Product  SaturateOnIntegerOverflow=on  InputSameDT=on
  Sum : Sum  Inputs=|+-  SaturateOnIntegerOverflow=on  InputSameDT=on
  Water Molar Mass : Gain  Gain=18.02e-3  SaturateOnIntegerOverflow=on
  n : Gain  Gain=fc_numberofcells  SaturateOnIntegerOverflow=on
  n/2F : Gain  Gain=fc_numberofcells/2/faradays  SaturateOnIntegerOverflow=on
  n/4F : Gain  Gain=fc_numberofcells/4/faradays  SaturateOnIntegerOverflow=on
  Mass Water Generated (kg/s) : Outport
  O2 Mass Reacted (kg/s) : Outport  Port=2
  Heat Produced (W) : Outport  Port=3
  Excess Ratio (lambda) : Outport  Port=4
  wires:
  Current/1 -> n/4F/1, n/2F/1, Product1/1
  n/2F/1 -> Water Molar Mass/1  "water produced mol/s"
  Water Molar Mass/1 -> Mass Water Generated (kg/s)/1  "mass water produced kg/sec"
  Stack Voltage/1 -> 1/n/1
  Ideal Cell Voltage/1 -> Sum/1
  1/n/1 -> Sum/2
  Sum/1 -> n/1
  n/1 -> Product1/2
  Product1/1 -> Heat Produced (W)/1
  Oxygen Molar Mass/1 -> Product/2, O2 Mass Reacted (kg/s)/1  "rate oxygen used kg/sec"
  n/4F/1 -> Oxygen Molar Mass/1  "rate oxygen used mol/sec"
  O2 mass flow in/1 -> Product/1  "Oxygen Mass Flow in (kg/s)"
  Product/1 -> Excess Ratio (lambda)/1

== system fcsystem/Fuel Cell Stack System/Stack/Cathode Mass Flow Model/Inlet Flow Properties to O2, N2 and Vapor Mass Flow ==
  note: Units
      | Pressure - Pascal, bar
      | Temperature - Kelvin
      | Voltage - Volt
      | Current - Ampere
      | Mass Flow - kg/sec
      | Rotational Speed - rad/sec
      | Power - Watt
      | humidity or relative humidity - 0 to 1
  Air Flow in : Inport
  1 - Total Mass Flow 2 - Temperature 3 - Pressure 4 - Relative Humidity 5 - Oxygen Mole Fraction (in Dry Air) : Demux  Outputs=5
  Constant1 : Constant  Value=vapormolarmass
  Constant2 : Constant
  Constant3 : Constant
  Dry Air Molar Mass : Fcn  Expr=u*oxygenmolarmass+(1-u)*nitrogenmolarmass
  Mole Fraction to Mass Fraction : Fcn  Expr=(u*oxygenmolarmass)/(u*oxygenmolarmass+(1-u)*nitrogenmolarmass)
  Product{2,6,8..9} (4 alike) : Product  SaturateOnIntegerOverflow=on  InputSameDT=on
  Product4 : Product  Inputs=*/  SaturateOnIntegerOverflow=on  InputSameDT=on
  Product5 : Product  Inputs=*/  SaturateOnIntegerOverflow=on  InputSameDT=on
  Product7 : Product  Inputs=*/  SaturateOnIntegerOverflow=on  InputSameDT=on
  Saturation Pressure (Pa) : Subsystem
  Sum4 : Sum  Inputs=-|+  SaturateOnIntegerOverflow=on  InputSameDT=on
  Sum5 : Sum  Inputs=++|  SaturateOnIntegerOverflow=on  InputSameDT=on
  Sum6 : Sum  Inputs=-+|  SaturateOnIntegerOverflow=on  InputSameDT=on
  Sum7 : Sum  Inputs=-|+  SaturateOnIntegerOverflow=on  InputSameDT=on
  Vapor Mass Flow in : Outport
  Oxygen Mass Flow in : Outport  Port=2
  Nitrogen Mass Flow in : Outport  Port=3
  wires:
  Saturation Pressure (Pa)/1(Saturation Pressure (Pa)) -> Product2/1
  Mole Fraction to Mass Fraction/1 -> Product8/2, Sum7/1  "Oxygen Mass Fraction"
  Air Flow in/1 -> 1 - Total Mass Flow 2 - Temperature 3 - Pressure 4 - Relative Humidity 5 - Oxygen Mole Fraction (in Dry Air)/1
  1 - Total Mass Flow 2 - Temperature 3 - Pressure 4 - Relative Humidity 5 - Oxygen Mole Fraction (in Dry Air)/2 -> Saturation Pressure (Pa)/1(Temperature (K))
  1 - Total Mass Flow 2 - Temperature 3 - Pressure 4 - Relative Humidity 5 - Oxygen Mole Fraction (in Dry Air)/3 -> Sum4/2
  Dry Air Molar Mass/1 -> Product4/2
  Constant1/1 -> Product4/1
  Product4/1 -> Product6/2
  1 - Total Mass Flow 2 - Temperature 3 - Pressure 4 - Relative Humidity 5 - Oxygen Mole Fraction (in Dry Air)/4 -> Product2/2
  Sum4/1 -> Product5/2  "dry air partial pressure"
  Product2/1 -> Sum4/1, Product5/1  "vapor partial pressure"
  Product5/1 -> Product6/1
  Sum5/1 -> Product7/2
  Product6/1 -> Sum5/2  "Humidity Ratio"
  Constant2/1 -> Sum5/1
  1 - Total Mass Flow 2 - Temperature 3 - Pressure 4 - Relative Humidity 5 - Oxygen Mole Fraction (in Dry Air)/1 -> Product7/1, Sum6/2
  Sum6/1 -> Vapor Mass Flow in/1  "vapor mass flow"
  1 - Total Mass Flow 2 - Temperature 3 - Pressure 4 - Relative Humidity 5 - Oxygen Mole Fraction (in Dry Air)/5 -> Dry Air Molar Mass/1, Mole Fraction to Mass Fraction/1
  Product7/1 -> Sum6/1, Product8/1, Product9/1  "dry air mass flow"
  Product8/1 -> Oxygen Mass Flow in/1  "Oxygen Mass Flow"
  Constant3/1 -> Sum7/2
  Sum7/1 -> Product9/2
  Product9/1 -> Nitrogen Mass Flow in/1  "Nitrogen Mass Flow"

== system fcsystem/Fuel Cell Stack System/Stack/Cathode Mass Flow Model/Nitrogen Balance ==
  N2 Mass Flow In (kg/s) : Inport
  N2 Mass Flow out (kg/s) : Inport  Port=2
  FC Temperature (K) : Inport  Port=3
  Initial Condition (kg) : Constant  Value=fcx0(3)
  Integrator : Integrator  InitialConditionSource=external
  Mux : Mux  Inputs=2
  Partial Pressure : Fcn  Expr=u[1]*nitrogengasconstant*u[2]/fc_cathode_volume
  Sum : Sum  Inputs=+-|  SaturateOnIntegerOverflow=on  InputSameDT=on
  N2 Mass (kg) : Outport
  N2 Partial Pressure : Outport  Port=2
  tag scope: mN2=global
  wires:
  Partial Pressure/1 -> N2 Partial Pressure/1
  Mux/1 -> Partial Pressure/1
  Integrator/1 -> Mux/1, N2 Mass (kg)/1, [mN2]
  FC Temperature (K)/1 -> Mux/2
  Initial Condition (kg)/1 -> Integrator/2
  Sum/1 -> Integrator/1
  N2 Mass Flow out (kg/s)/1 -> Sum/2
  N2 Mass Flow In (kg/s)/1 -> Sum/1

== system fcsystem/Fuel Cell Stack System/Stack/Cathode Mass Flow Model/Outlet Flow Properties to O2, N2 and Vapor Mass Flow ==
  note: Units
      | Pressure - Pascal, bar
      | Temperature - Kelvin
      | Voltage - Volt
      | Current - Ampere
      | Mass Flow - kg/sec
      | Rotational Speed - rad/sec
      | Power - Watt
      | humidity or relative humidity - 0 to 1
  Air Flow out : Inport
  1 - Total Mass Flow 2 - Temperature 3 - Pressure 4 - Relative Humidity 5 - Oxygen Mole Fraction (in Dry Air) : Demux  Outputs=5
  Constant1 : Constant  Value=vapormolarmass
  Constant2 : Constant
  Constant3 : Constant
  Dry Air Molar Mass : Fcn  Expr=u*oxygenmolarmass+(1-u)*nitrogenmolarmass
  Mole Fraction to Mass Fraction : Fcn  Expr=(u*oxygenmolarmass)/(u*oxygenmolarmass+(1-u)*nitrogenmolarmass)
  Product{2,6,8..9} (4 alike) : Product  SaturateOnIntegerOverflow=on  InputSameDT=on
  Product4 : Product  Inputs=*/  SaturateOnIntegerOverflow=on  InputSameDT=on
  Product5 : Product  Inputs=*/  SaturateOnIntegerOverflow=on  InputSameDT=on
  Product7 : Product  Inputs=*/  SaturateOnIntegerOverflow=on  InputSameDT=on
  Saturation Pressure (Pa) : Subsystem
  Sum4 : Sum  Inputs=-|+  SaturateOnIntegerOverflow=on  InputSameDT=on
  Sum5 : Sum  Inputs=++|  SaturateOnIntegerOverflow=on  InputSameDT=on
  Sum6 : Sum  Inputs=-+|  SaturateOnIntegerOverflow=on  InputSameDT=on
  Sum7 : Sum  Inputs=-|+  SaturateOnIntegerOverflow=on  InputSameDT=on
  Vapor Mass Flow out : Outport
  Oxygen Mass Flow out : Outport  Port=2
  Nitrogen Mass Flow out : Outport  Port=3
  wires:
  Product9/1 -> Nitrogen Mass Flow out/1  "Nitrogen Mass Flow"
  Sum7/1 -> Product9/2
  Constant3/1 -> Sum7/2
  Mole Fraction to Mass Fraction/1 -> Sum7/1, Product8/2  "Oxygen Mass Fraction"
  Product8/1 -> Oxygen Mass Flow out/1  "Oxygen Mass Flow"
  Product7/1 -> Product9/1, Product8/1, Sum6/1  "dry air mass flow"
  1 - Total Mass Flow 2 - Temperature 3 - Pressure 4 - Relative Humidity 5 - Oxygen Mole Fraction (in Dry Air)/5 -> Mole Fraction to Mass Fraction/1, Dry Air Molar Mass/1
  Sum6/1 -> Vapor Mass Flow out/1  "vapor mass flow"
  1 - Total Mass Flow 2 - Temperature 3 - Pressure 4 - Relative Humidity 5 - Oxygen Mole Fraction (in Dry Air)/1 -> Sum6/2, Product7/1
  Constant2/1 -> Sum5/1
  Product6/1 -> Sum5/2  "Humidity Ratio"
  Sum5/1 -> Product7/2
  Product5/1 -> Product6/1
  Product2/1 -> Product5/1, Sum4/1  "vapor partial pressure"
  Sum4/1 -> Product5/2  "dry air partial pressure"
  1 - Total Mass Flow 2 - Temperature 3 - Pressure 4 - Relative Humidity 5 - Oxygen Mole Fraction (in Dry Air)/4 -> Product2/2
  Saturation Pressure (Pa)/1(Saturation Pressure (Pa)) -> Product2/1
  Product4/1 -> Product6/2
  Constant1/1 -> Product4/1
  Dry Air Molar Mass/1 -> Product4/2
  1 - Total Mass Flow 2 - Temperature 3 - Pressure 4 - Relative Humidity 5 - Oxygen Mole Fraction (in Dry Air)/3 -> Sum4/2
  1 - Total Mass Flow 2 - Temperature 3 - Pressure 4 - Relative Humidity 5 - Oxygen Mole Fraction (in Dry Air)/2 -> Saturation Pressure (Pa)/1(Temperature (K))
  Air Flow out/1 -> 1 - Total Mass Flow 2 - Temperature 3 - Pressure 4 - Relative Humidity 5 - Oxygen Mole Fraction (in Dry Air)/1

== system fcsystem/Fuel Cell Stack System/Stack/Cathode Mass Flow Model/Oxygen Balance ==
  O2 Mass Flow In (kg/s) : Inport
  O2 Mass Flow out (kg/s) : Inport  Port=2
  O2 Mass reacted (kg/s) : Inport  Port=3
  FC Temperature (K) : Inport  Port=4
  Initial Condition (kg) : Constant  Value=fcx0(1)
  Integrator : Integrator  InitialConditionSource=external
  Mux : Mux  Inputs=2
  Partial Pressure : Fcn  Expr=u[1]*oxygengasconstant*u[2]/fc_cathode_volume
  Sum : Sum  Inputs=+--  SaturateOnIntegerOverflow=on  InputSameDT=on
  O2 Mass (kg) : Outport
  O2 Partial Pressure : Outport  Port=2
  tag scope: mO2=global
  wires:
  O2 Mass Flow In (kg/s)/1 -> Sum/1
  O2 Mass Flow out (kg/s)/1 -> Sum/2
  O2 Mass reacted (kg/s)/1 -> Sum/3
  Sum/1 -> Integrator/1
  Initial Condition (kg)/1 -> Integrator/2
  FC Temperature (K)/1 -> Mux/2
  Integrator/1 -> O2 Mass (kg)/1, Mux/1, [mO2]
  Mux/1 -> Partial Pressure/1
  Partial Pressure/1 -> O2 Partial Pressure/1

== system fcsystem/Fuel Cell Stack System/Stack/Cathode Mass Flow Model/Pressure Calculation ==
  O2 Partial Pressure : Inport
  N2 Partial Pressure : Inport  Port=2
  Vapor Partial Pressure : Inport  Port=3
  Product : Product  Inputs=*/  SaturateOnIntegerOverflow=on  InputSameDT=on
  Sum : Sum  Inputs=+|+  SaturateOnIntegerOverflow=on  InputSameDT=on
  Sum1 : Sum  Inputs=+|+  SaturateOnIntegerOverflow=on  InputSameDT=on
  Cathode Pressure : Outport
  O2 Mole Fraction : Outport  Port=2
  wires:
  N2 Partial Pressure/1 -> Sum/2
  O2 Partial Pressure/1 -> Sum/1, Product/1
  Product/1 -> O2 Mole Fraction/1  "O2 Mole Fraction"
  Sum/1 -> Product/2, Sum1/1  "Dry Air Partial Pressure"
  Vapor Partial Pressure/1 -> Sum1/2
  Sum1/1 -> Cathode Pressure/1  "Total Pressure"

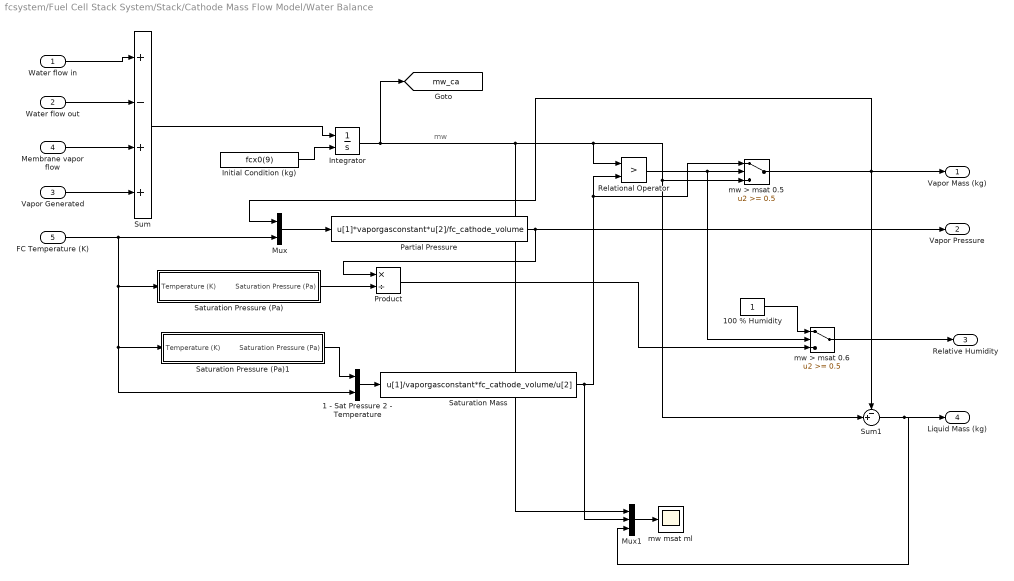
== system fcsystem/Fuel Cell Stack System/Stack/Cathode Mass Flow Model/Water Balance ==
  note: mw
  Water flow in : Inport
  Water flow out : Inport  Port=2
  Vapor Generated : Inport  Port=3
  Membrane vapor flow : Inport  Port=4
  FC Temperature (K) : Inport  Port=5
  1 - Sat Pressure 2 - Temperature : Mux  Inputs=2
  100 % Humidity : Constant
  Initial Condition (kg) : Constant  Value=fcx0(9)
  Integrator : Integrator  InitialConditionSource=external
  Mux : Mux  Inputs=2
  Mux1 : Mux  Inputs=3
  Partial Pressure : Fcn  Expr=u[1]*vaporgasconstant*u[2]/fc_cathode_volume
  Product : Product  Inputs=*/  SaturateOnIntegerOverflow=on  InputSameDT=on
  Relational Operator : RelationalOperator  Operator=>  InputSameDT=on
  Saturation Mass : Fcn  Expr=u[1]/vaporgasconstant*fc_cathode_volume/u[2]
  Saturation Pressure (Pa) : Subsystem
  Saturation Pressure (Pa)1 : Subsystem
  Sum : Sum  Inputs=+-++  SaturateOnIntegerOverflow=on  InputSameDT=on
  Sum1 : Sum  Inputs=-+|  SaturateOnIntegerOverflow=on  InputSameDT=on
  mw msat ml : Scope
      settings: SaveName=ScopeData4
  mw > msat 0.5 : Switch  Threshold=0.5  SaturateOnIntegerOverflow=on  InputSameDT=on
  mw > msat 0.6 : Switch  Threshold=0.5  SaturateOnIntegerOverflow=on  InputSameDT=on
  Vapor Mass (kg) : Outport
  Vapor Pressure : Outport  Port=2
  Relative Humidity : Outport  Port=3
  Liquid Mass (kg) : Outport  Port=4
  tag scope: mw_ca=global
  wires:
  Water flow in/1 -> Sum/1
  Water flow out/1 -> Sum/2
  Membrane vapor flow/1 -> Sum/3
  FC Temperature (K)/1 -> Mux/2, Saturation Pressure (Pa)/1(Temperature (K)), 1 - Sat Pressure 2 - Temperature/2, Saturation Pressure (Pa)1/1(Temperature (K))
  Integrator/1 -> [mw_ca], Relational Operator/1, mw > msat 0.5/3, Sum1/2, Mux1/1
  Initial Condition (kg)/1 -> Integrator/2
  Saturation Pressure (Pa)/1(Saturation Pressure (Pa)) -> Product/2
  Partial Pressure/1 -> Product/1, Vapor Pressure/1
  Mux/1 -> Partial Pressure/1
  Saturation Pressure (Pa)1/1(Saturation Pressure (Pa)) -> 1 - Sat Pressure 2 - Temperature/1
  1 - Sat Pressure 2 - Temperature/1 -> Saturation Mass/1
  Saturation Mass/1 -> Relational Operator/2, mw > msat 0.5/1, Mux1/2
  100 % Humidity/1 -> mw > msat 0.6/1
  Product/1 -> mw > msat 0.6/3
  mw > msat 0.6/1 -> Relative Humidity/1
  mw > msat 0.5/1 -> Mux/1, Sum1/1, Vapor Mass (kg)/1
  Relational Operator/1 -> mw > msat 0.5/2, mw > msat 0.6/2
  Sum1/1 -> Liquid Mass (kg)/1, Mux1/3
  Sum/1 -> Integrator/1
  Vapor Generated/1 -> Sum/4
  Mux1/1 -> mw msat ml/1

== system fcsystem/Fuel Cell Stack System/Stack/Stack Voltage Model/Saturation Pressure (Pa) ==
  Temperature (K) : Inport
  333.15K : Switch  Threshold=333.15  SaturateOnIntegerOverflow=on  InputSameDT=on
  433.15K : Switch  Threshold=433.15  SaturateOnIntegerOverflow=on  InputSameDT=on
  533.15K : Switch  SaturateOnIntegerOverflow=on  InputSameDT=on
  Water Sat. Pressure in kPa (using 4th order approx) 333.15K<t<433.15K : Fcn  Expr=1.508306069874139e-006*u^4-0.00184416225407*u^3+0.85777718452468*u^2-1.796665242102233e+002*u+1.428163901107325e+004
  Water Sat. Pressure in kPa (using 4th order approx) 433.15<t<533.15 : Fcn  Expr=1.338811201296496e-006*u^4-0.00154136533415*u^3+0.65477998701526*u^2-1.191331991860853e+002*u+7.506492157825003e+003
  Water Sat. Pressure in kPa (using 4th order approx) t<333.15K : Fcn  Expr=6.853193243616891e-007*u^4-7.432459524835483e-004*u^3+0.30413751828818*u^2-55.61363113326989*u+3.831800671740628e+003
  Water Sat. Pressure in kPa (using 4th order approx) t>533.15K : Fcn  Expr=1.648503329422670e-6*u^4-0.00209262218193*u^3+1.01793196387371*u^2-2.241752317908023e2*u+1.878246444328017e4
  kPa to Pa : Gain  Gain=1000  SaturateOnIntegerOverflow=on
  Saturation Pressure (Pa) : Outport
  wires:
  Temperature (K)/1 -> Water Sat. Pressure in kPa (using 4th order approx) t>533.15K/1, Water Sat. Pressure in kPa (using 4th order approx) 433.15<t<533.15/1, Water Sat. Pressure in kPa (using 4th order approx) 333.15K<t<433.15K/1, Water Sat. Pressure in kPa (using 4th order approx) t<333.15K/1, 533.15K/2, 433.15K/2, 333.15K/2
  533.15K/1 -> kPa to Pa/1
  kPa to Pa/1 -> Saturation Pressure (Pa)/1
  433.15K/1 -> 533.15K/3
  Water Sat. Pressure in kPa (using 4th order approx) t>533.15K/1 -> 533.15K/1
  Water Sat. Pressure in kPa (using 4th order approx) 433.15<t<533.15/1 -> 433.15K/1
  333.15K/1 -> 433.15K/3
  Water Sat. Pressure in kPa (using 4th order approx) 333.15K<t<433.15K/1 -> 333.15K/1
  Water Sat. Pressure in kPa (using 4th order approx) t<333.15K/1 -> 333.15K/3

== system fcsystem/Fuel Cell Stack System/Compressor/Compressor/Calculate Humidity Change/Saturation Pressure (Pa) ==
  Temperature (K) : Inport
  333.15K : Switch  Threshold=333.15  SaturateOnIntegerOverflow=on  InputSameDT=on
  433.15K : Switch  Threshold=433.15  SaturateOnIntegerOverflow=on  InputSameDT=on
  533.15K : Switch  Threshold=533.15  SaturateOnIntegerOverflow=on  InputSameDT=on
  Water Sat. Pressure in kPa (using 4th order approx) 333.15K<t<433.15K : Fcn  Expr=1.508306069874139e-006*u^4-0.00184416225407*u^3+0.85777718452468*u^2-1.796665242102233e+002*u+1.428163901107325e+004
  Water Sat. Pressure in kPa (using 4th order approx) 433.15<t<533.15 : Fcn  Expr=1.338811201296496e-006*u^4-0.00154136533415*u^3+0.65477998701526*u^2-1.191331991860853e+002*u+7.506492157825003e+003
  Water Sat. Pressure in kPa (using 4th order approx) t<333.15K : Fcn  Expr=6.853193243616891e-007*u^4-7.432459524835483e-004*u^3+0.30413751828818*u^2-55.61363113326989*u+3.831800671740628e+003
  Water Sat. Pressure in kPa (using 4th order approx) t>533.15K : Fcn  Expr=1.648503329422670e-6*u^4-0.00209262218193*u^3+1.01793196387371*u^2-2.241752317908023e2*u+1.878246444328017e4
  kPa to Pa : Gain  Gain=1000  SaturateOnIntegerOverflow=on
  Saturation Pressure (Pa) : Outport
  wires:
  Water Sat. Pressure in kPa (using 4th order approx) t<333.15K/1 -> 333.15K/3
  Water Sat. Pressure in kPa (using 4th order approx) 333.15K<t<433.15K/1 -> 333.15K/1
  333.15K/1 -> 433.15K/3
  Water Sat. Pressure in kPa (using 4th order approx) 433.15<t<533.15/1 -> 433.15K/1
  Water Sat. Pressure in kPa (using 4th order approx) t>533.15K/1 -> 533.15K/1
  433.15K/1 -> 533.15K/3
  kPa to Pa/1 -> Saturation Pressure (Pa)/1
  533.15K/1 -> kPa to Pa/1
  Temperature (K)/1 -> 333.15K/2, 433.15K/2, 533.15K/2, Water Sat. Pressure in kPa (using 4th order approx) t<333.15K/1, Water Sat. Pressure in kPa (using 4th order approx) 333.15K<t<433.15K/1, Water Sat. Pressure in kPa (using 4th order approx) 433.15<t<533.15/1, Water Sat. Pressure in kPa (using 4th order approx) t>533.15K/1
